simulink model "k1vissr2t"  (Simulink 8.8)
settings: Solver=VariableStepAuto  StartTime=0.0  StopTime=10.0  RelTol=1e-3  EnableMultiTasking=on
libraries: cdsIPCx x10, cdsFilt x4, cdsCDO64 x3, cdsCDI64 x2, dac x2, TYPEB_MASTER x2, cdsAdcx0 x1, TOWER_MASTER x1, cdsParameters x1
settings Model: SuppressorTable=22 serialization::archive 11 0 3 0 0 0 11 0  Creator=controls  LastModifiedBy=controls
settings DataIOCC: SaveFormat=Dataset  SignalLoggingSaveFormat=Dataset
settings DebuggingCC: UnderspecifiedInitializationDetection=Simplified  MergeDetectMultiDrivingBlocksExec=error  FcnCallInpInsideContextMsg=error  AllowSymbolicDim=off  StateNameClashWarn=none
settings HardwareCC: ProdBitPerPointer=64  ProdBitPerSizeT=64  ProdBitPerPtrDiffT=64  ProdLargestAtomicFloat=Float  ProdIntDivRoundTo=Zero  ProdEndianess=LittleEndian  ProdWordSize=64  ProdHWDeviceType=Intel->x86-64 (Windows64)
settings GRTTargetCC: GeneratePreprocessorConditionals=Use local settings  CombineOutputUpdateFcns=on  GRTInterface=off

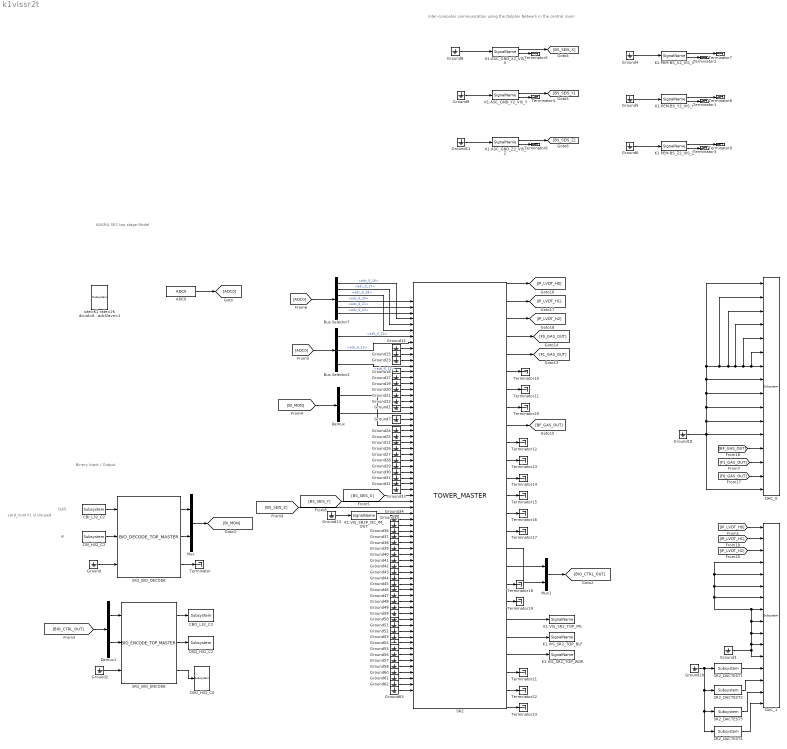
== system k1vissr2t ==
  note: KAGRA SR2 top stage Model
  note: Binary Input / Output
  note: card_num=1 is Unused
  note: GAS
  note: IP
  note: Inter-computer communication using
      | the Dolphin Network in the central room
  ADC0 : cdsAdcx0/ADC0  Tag=cdsAdc  Description=|
      | type-GSC_16AI64SSA
      | card_num=0
      settings: AttributesFormatString=%<Description>\n%<Tag>
  Bus Selector2 : BusSelector  Description=ADC Selector  OutputSignals=adc_0_14,adc_0_13,adc_0_12
      settings: AttributesFormatString=%<Description>
  Bus Selector7 : BusSelector  Description=ADC Selector  OutputSignals=adc_0_16,adc_0_17,adc_0_18,adc_0_20,adc_0_21,adc_0_22
      settings: AttributesFormatString=%<Description>
  CBI_H32_C2 : cdsCDI64/Subsystem  Tag=cdsCDI64  Description=card_num=5
      settings: AttributesFormatString=%<Tag>\n%<Description>
  CBI_L32_C2 : cdsCDI64/Subsystem  Tag=cdsCDI64  Description=card_num=4
      settings: AttributesFormatString=%<Tag>\n%<Description>
  CBO_H32_C0 : cdsCDO64/Subsystem  Tag=cdsCDO64  Description=card_num=1
      settings: AttributesFormatString=%<Tag>\n%<Description>
  CBO_H32_C2 : cdsCDO64/Subsystem  Tag=cdsCDO64  Description=card_num=5
      settings: AttributesFormatString=%<Tag>\n%<Description>
  CBO_L32_C2 : cdsCDO64/Subsystem  Tag=cdsCDO64  Description=card_num=4
      settings: AttributesFormatString=%<Tag>\n%<Description>
  DAC_0 : dac/Subsystem  Description=|
      | type=GSC_16AO16,
      | card_num=0
      settings: AttributesFormatString=%<Description>
  DAC_1 : dac/Subsystem  Description=|
      | type=GSC_16AO16,
      | card_num=1
      settings: AttributesFormatString=%<Description>
  Demux : Demux  Outputs=2
  Demux1 : Demux  Outputs=2
  Ground{,1..63} (64 alike) : Ground
  K1:ASC_GND_X2_VIS_X : cdsIPCx/SignalName  Tag=cdsIPCx_PCIE  Description=Inter-Process Communication via PCI Express network.
      settings: AttributesFormatString=%<Tag>
  K1:ASC_GND_Y2_VIS_Y : cdsIPCx/SignalName  Tag=cdsIPCx_PCIE  Description=Inter-Process Communication via PCI Express network.
      settings: AttributesFormatString=%<Tag>
  K1:ASC_GND_Z2_VIS_Z : cdsIPCx/SignalName  Tag=cdsIPCx_PCIE  Description=Inter-Process Communication via PCI Express network.
      settings: AttributesFormatString=%<Tag>
  K1:PEM-BS_X2_VIS_X : cdsIPCx/SignalName  Tag=cdsIPCx_PCIE  Description=Inter-Process Communication via PCI Express network.
      settings: AttributesFormatString=%<Tag>
  K1:PEM-BS_Y2_VIS_Y : cdsIPCx/SignalName  Tag=cdsIPCx_PCIE  Description=Inter-Process Communication via PCI Express network.
      settings: AttributesFormatString=%<Tag>
  K1:PEM-BS_Z2_VIS_Z : cdsIPCx/SignalName  Tag=cdsIPCx_PCIE  Description=Inter-Process Communication via PCI Express network.
      settings: AttributesFormatString=%<Tag>
  K1:VIS_SR2P_ISC_IM_OUT : cdsIPCx/SignalName  Tag=cdsIPCx_SHMEM  Description=Inter-Process Communication via Shared memory.
      settings: AttributesFormatString=%<Tag>
  K1:VIS_SR2_TOP_BLF : cdsIPCx/SignalName  Tag=cdsIPCx_SHMEM  Description=Inter-Process Communication via Shared memory.
      settings: AttributesFormatString=%<Tag>
  K1:VIS_SR2_TOP_MS : cdsIPCx/SignalName  Tag=cdsIPCx_SHMEM  Description=Inter-Process Communication via Shared memory.
      settings: AttributesFormatString=%<Tag>
  K1:VIS_SR2_TOP_WDR : cdsIPCx/SignalName  Tag=cdsIPCx_SHMEM  Description=Inter-Process Communication via Shared memory.
      settings: AttributesFormatString=%<Tag>
  Mux : Mux  Inputs=2
  Mux1 : Mux  Inputs=2
  SR2 : TOWER_MASTER/TOWER_MASTER
  SR2_BIO_DECODE : TYPEB_MASTER/BIO_DECODE_TOP_MASTER
  SR2_BIO_ENCODE : TYPEB_MASTER/BIO_ENCODE_TOP_MASTER
  SR2_DACTEST1 : cdsFilt/Subsystem  Tag=cdsFilt  Description=|
      | Purpose:                                                                                                                                                                                                                                  
      | Standard CDS IIR filter module.                                                                                                                                                                                                           
      |                                                                                                                                                                                                                                           
      | Operation:                                                                                                                                                                                                                                
      | Consists of 10 second order section IIR filters, plus a ramped gain stage. In FE code, also provides pre-defined test points and excitation channel inputs. The filter coefficients are defined in the LIGO system using the 'foton' tool.
      |                                                                                                                                                                                                                                           
      | Usage:                                                                                                                                                                                                                                    
      | Name the part with the desired filter module name.
      settings: AttributesFormatString=%<Tag>
  SR2_DACTEST2 : cdsFilt/Subsystem  Tag=cdsFilt  Description=|
      | Purpose:                                                                                                                                                                                                                                  
      | Standard CDS IIR filter module.                                                                                                                                                                                                           
      |                                                                                                                                                                                                                                           
      | Operation:                                                                                                                                                                                                                                
      | Consists of 10 second order section IIR filters, plus a ramped gain stage. In FE code, also provides pre-defined test points and excitation channel inputs. The filter coefficients are defined in the LIGO system using the 'foton' tool.
      |                                                                                                                                                                                                                                           
      | Usage:                                                                                                                                                                                                                                    
      | Name the part with the desired filter module name.
      settings: AttributesFormatString=%<Tag>
  SR2_DACTEST3 : cdsFilt/Subsystem  Tag=cdsFilt  Description=|
      | Purpose:                                                                                                                                                                                                                                  
      | Standard CDS IIR filter module.                                                                                                                                                                                                           
      |                                                                                                                                                                                                                                           
      | Operation:                                                                                                                                                                                                                                
      | Consists of 10 second order section IIR filters, plus a ramped gain stage. In FE code, also provides pre-defined test points and excitation channel inputs. The filter coefficients are defined in the LIGO system using the 'foton' tool.
      |                                                                                                                                                                                                                                           
      | Usage:                                                                                                                                                                                                                                    
      | Name the part with the desired filter module name.
      settings: AttributesFormatString=%<Tag>
  SR2_DACTEST4 : cdsFilt/Subsystem  Tag=cdsFilt  Description=|
      | Purpose:                                                                                                                                                                                                                                  
      | Standard CDS IIR filter module.                                                                                                                                                                                                           
      |                                                                                                                                                                                                                                           
      | Operation:                                                                                                                                                                                                                                
      | Consists of 10 second order section IIR filters, plus a ramped gain stage. In FE code, also provides pre-defined test points and excitation channel inputs. The filter coefficients are defined in the LIGO system using the 'foton' tool.
      |                                                                                                                                                                                                                                           
      | Usage:                                                                                                                                                                                                                                    
      | Name the part with the desired filter module name.
      settings: AttributesFormatString=%<Tag>
  Terminator{,1..23} (24 alike) : Terminator
  site=K1 rate=2K dcuid=65 host=k1sr2 specific_cpu=2 adcSlave=1 : cdsParameters/Subsystem  Tag=cdsParameters  Description=|
      | Purpose:                                                                                                                                                                                                                                
      | Provide system parameters to the FE code generator to properly configure the generated EPICS names, rep rate of the FE controller, and the Data Acquisition node ID for proper storage of data from this FE controller.                 
      |                                                                                                                                                                                                                                         
      | Useage:                                                                                                                                                                                                                                 
      | The part NAME field is used to identify the FE parameters. It must be of the form:                                                                                                                                                      
      | site=                                                                                                                                                                                                                                   
      | rate=                                                                                                                                                                                                                                   
      | dcuid=                                                                                                                                                                                                                                  
      |                                                                                                                                                                                                                                         
      | Where:                                                                                                                                                                                                                                  
      | site= argument may be H1, H2, L1, M1, G1, either as a single argument or multiple, for example site=H1,H2. These are the only names allowed. These will become the first two characters of all EPICS and signal names (for example G1:).
      |                                                                                                                                                                                                                                         
      | rate= may be 2K, 16K, 32K, or 64K                                                                                                                                                                                                       
      |                                                                                                                                                                                                                                         
      | dcuid= is site specific ie it must be unique at each site.
      settings: AttributesFormatString=%<Tag>
  wires:
  SR2/4 -> [F0_GAS_OUT]
  SR2/5 -> [F1_GAS_OUT]
  SR2/9 -> [BF_GAS_OUT]
  ADC0/1 -> [ADC0]
  [ADC0] -> Bus Selector7/1
  [ADC0] -> Bus Selector2/1
  Bus Selector2/2 -> SR2/8  "<adc_0_13>"
  Bus Selector2/3 -> SR2/12  "<adc_0_12>"
  Bus Selector7/1 -> SR2/4  "<adc_0_16>"
  Bus Selector7/2 -> SR2/5  "<adc_0_17>"
  Bus Selector7/3 -> SR2/6  "<adc_0_18>"
  Ground7/1 -> SR2/21
  SR2_BIO_ENCODE/1 -> CBO_L32_C2/1
  CBI_L32_C2/1 -> SR2_BIO_DECODE/1
  SR2_BIO_DECODE/1 -> Mux/1
  SR2_BIO_DECODE/2 -> Mux/2
  Mux/1 -> [BI_MON]
  [BI_MON] -> Demux/1
  Ground1/1 -> SR2/19
  Mux1/1 -> [BIO_CTRL_OUT]
  SR2/17 -> Mux1/1
  [BIO_CTRL_OUT] -> Demux1/1
  CBI_H32_C2/1 -> SR2_BIO_DECODE/2
  SR2_BIO_ENCODE/2 -> CBO_H32_C2/1
  [F1_GAS_OUT] -> DAC_0/14
  [F0_GAS_OUT] -> DAC_0/15
  [BF_GAS_OUT] -> DAC_0/13
  SR2/2 -> [IP_LVDT_H1]
  SR2/1 -> [IP_LVDT_H0]
  SR2/3 -> [IP_LVDT_H2]
  [IP_LVDT_H0] -> DAC_1/1
  [IP_LVDT_H1] -> DAC_1/2
  [IP_LVDT_H2] -> DAC_1/3
  Bus Selector2/1 -> SR2/7  "<adc_0_14>"
  Ground18/1 -> DAC_0/11, DAC_0/10, DAC_0/9, DAC_0/1, DAC_0/2, DAC_0/3, DAC_0/4, DAC_0/5, DAC_0/6, DAC_0/7, DAC_0/8, DAC_0/16, DAC_0/12
  Ground3/1 -> DAC_1/12, DAC_1/7, DAC_1/6, DAC_1/5, DAC_1/4, DAC_1/8, DAC_1/9, DAC_1/10, DAC_1/11
  SR2_DACTEST3/1 -> DAC_1/15
  SR2_DACTEST4/1 -> DAC_1/16
  SR2_DACTEST2/1 -> DAC_1/14
  SR2_DACTEST1/1 -> DAC_1/13
  Ground10/1 -> SR2_DACTEST4/1, SR2_DACTEST3/1, SR2_DACTEST2/1, SR2_DACTEST1/1
  Demux1/2 -> SR2_BIO_ENCODE/2
  SR2/20 -> K1:VIS_SR2_TOP_MS/1
  SR2/22 -> K1:VIS_SR2_TOP_WDR/1
  Ground/1 -> SR2_BIO_DECODE/3
  SR2_BIO_DECODE/3 -> Terminator/1
  Demux1/1 -> SR2_BIO_ENCODE/1
  SR2_BIO_ENCODE/3 -> CBO_H32_C0/1
  Ground2/1 -> SR2_BIO_ENCODE/3
  SR2/16 -> Mux1/2
  SR2/21 -> K1:VIS_SR2_TOP_BLF/1
  Ground4/1 -> K1:PEM-BS_X2_VIS_X/1
  Ground5/1 -> K1:PEM-BS_Y2_VIS_Y/1
  Ground6/1 -> K1:PEM-BS_Z2_VIS_Z/1
  K1:PEM-BS_X2_VIS_X/1 -> Terminator7/1
  K1:PEM-BS_Y2_VIS_Y/1 -> Terminator8/1
  K1:PEM-BS_Z2_VIS_Z/1 -> Terminator9/1
  K1:PEM-BS_X2_VIS_X/2 -> Terminator2/1
  K1:PEM-BS_Y2_VIS_Y/2 -> Terminator1/1
  K1:PEM-BS_Z2_VIS_Z/2 -> Terminator3/1
  [BS_SEIS_X] -> SR2/34
  [BS_SEIS_Z] -> SR2/36
  [BS_SEIS_Y] -> SR2/35
  Ground8/1 -> K1:ASC_GND_X2_VIS_X/1
  Ground9/1 -> K1:ASC_GND_Y2_VIS_Y/1
  Ground11/1 -> K1:ASC_GND_Z2_VIS_Z/1
  K1:ASC_GND_X2_VIS_X/1 -> [BS_SEIS_X]
  K1:ASC_GND_Y2_VIS_Y/1 -> [BS_SEIS_Y]
  K1:ASC_GND_Z2_VIS_Z/1 -> [BS_SEIS_Z]
  K1:ASC_GND_X2_VIS_X/2 -> Terminator5/1
  K1:ASC_GND_Y2_VIS_Y/2 -> Terminator4/1
  K1:ASC_GND_Z2_VIS_Z/2 -> Terminator6/1
  Ground13/1 -> K1:VIS_SR2P_ISC_IM_OUT/1
  K1:VIS_SR2P_ISC_IM_OUT/1 -> SR2/37
  Demux/1 -> SR2/22
  Demux/2 -> SR2/20
  Ground14/1 -> SR2/9
  Ground15/1 -> SR2/10
  Ground16/1 -> SR2/13
  Ground17/1 -> SR2/14
  Ground19/1 -> SR2/15
  Ground20/1 -> SR2/16
  Ground21/1 -> SR2/17
  Ground22/1 -> SR2/18
  Ground24/1 -> SR2/23
  Ground25/1 -> SR2/24
  Ground12/1 -> SR2/25
  Ground26/1 -> SR2/26
  Ground27/1 -> SR2/27
  Ground28/1 -> SR2/28
  Ground29/1 -> SR2/29
  Ground30/1 -> SR2/30
  Ground31/1 -> SR2/31
  Ground32/1 -> SR2/32
  Ground33/1 -> SR2/33
  Ground34/1 -> SR2/38
  Ground35/1 -> SR2/39
  Ground36/1 -> SR2/40
  Ground37/1 -> SR2/41
  Ground38/1 -> SR2/42
  Ground39/1 -> SR2/43
  Ground40/1 -> SR2/44
  Ground41/1 -> SR2/45
  Ground42/1 -> SR2/46
  Ground43/1 -> SR2/47
  Ground44/1 -> SR2/48
  Ground45/1 -> SR2/49
  Ground46/1 -> SR2/50
  Ground47/1 -> SR2/51
  Ground48/1 -> SR2/52
  Ground49/1 -> SR2/53
  Ground50/1 -> SR2/55
  Ground51/1 -> SR2/56
  Ground52/1 -> SR2/57
  Ground53/1 -> SR2/58
  Ground54/1 -> SR2/59
  Ground55/1 -> SR2/60
  Ground56/1 -> SR2/61
  Ground57/1 -> SR2/62
  Ground58/1 -> SR2/63
  SR2/18 -> Terminator18/1
  SR2/19 -> Terminator19/1
  SR2/10 -> Terminator12/1
  SR2/11 -> Terminator13/1
  SR2/12 -> Terminator14/1
  SR2/13 -> Terminator15/1
  SR2/14 -> Terminator16/1
  SR2/15 -> Terminator17/1
  SR2/6 -> Terminator10/1
  SR2/7 -> Terminator11/1
  Bus Selector7/4 -> SR2/1  "<adc_0_20>"
  Bus Selector7/5 -> SR2/2  "<adc_0_21>"
  Bus Selector7/6 -> SR2/3  "<adc_0_22>"
  Ground23/1 -> SR2/11
  SR2/8 -> Terminator20/1
  Ground59/1 -> SR2/54
  Ground62/1 -> SR2/66
  Ground61/1 -> SR2/65
  Ground60/1 -> SR2/64
  SR2/24 -> Terminator22/1
  SR2/23 -> Terminator21/1
  SR2/25 -> Terminator23/1
  Ground63/1 -> SR2/67
